simulink model "CH01"  (R2024b)
settings: Solver=FixedStepAuto  StartTime=0.0  StopTime=10  FixedStep=0.001  RelTol=1e-3
settings Model: Creator=headl  LastModifiedBy=headl

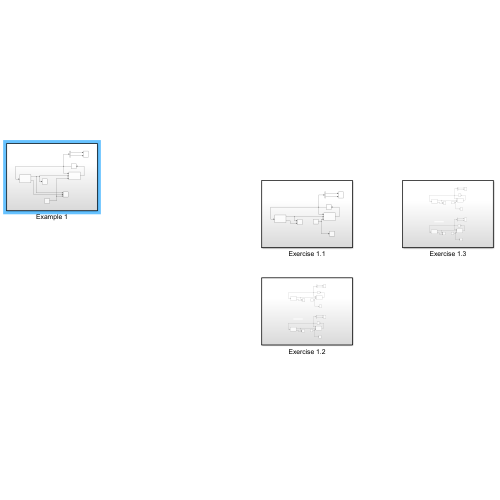
[thumbnail: Simulink's stored preview of the top-level diagram]
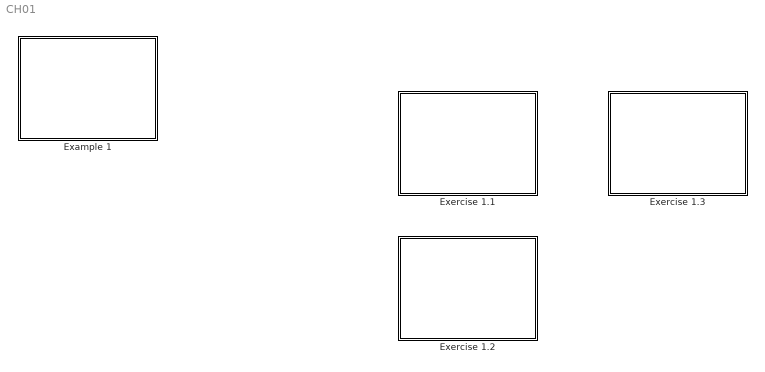
== system CH01 ==
  Example 1 : Subsystem
  Exercise 1.1 : Subsystem
  Exercise 1.2 : Subsystem
  Exercise 1.3 : Subsystem

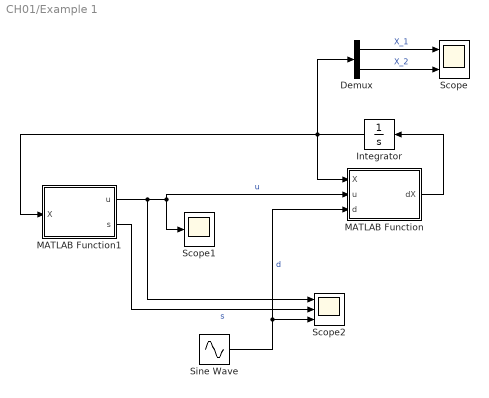
== system CH01/Example 1 ==
  Demux : Demux  Outputs=2
  Integrator : Integrator  InitialCondition=[3;0.4]
  MATLAB Function : MATLAB Function  TreatAsAtomicUnit=on
  MATLAB Function1 : MATLAB Function  TreatAsAtomicUnit=on
  Scope : Scope  NumInputPorts=2
  Scope1 : Scope
  Scope2 : Scope  NumInputPorts=3
  Sine Wave : Sin  Amplitude=0.8  Frequency=4  SampleTime=0
  wires:
  MATLAB Function/1(dX) -> Integrator/1
  Integrator/1 -> Demux/1, MATLAB Function/1(X), MATLAB Function1/1(X)
  Demux/2 -> Scope/2  "X_2"
  MATLAB Function1/1(u) -> Scope2/1, Scope1/1, MATLAB Function/2(u)  "u"
  Demux/1 -> Scope/1  "X_1"
  MATLAB Function1/2(s) -> Scope2/2  "s"
  Sine Wave/1 -> MATLAB Function/3(d), Scope2/3  "d"

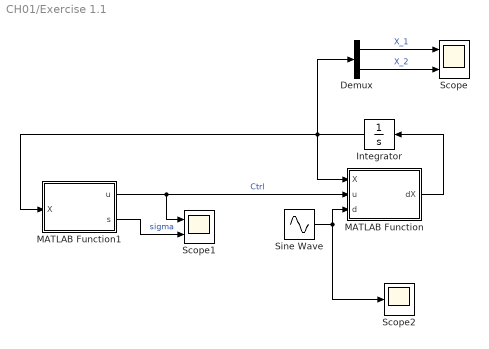
== system CH01/Exercise 1.1 ==
  Demux : Demux  Outputs=2
  Integrator : Integrator  InitialCondition=[2;0.5]
  MATLAB Function : MATLAB Function  TreatAsAtomicUnit=on
  MATLAB Function1 : MATLAB Function  TreatAsAtomicUnit=on
  Scope : Scope  NumInputPorts=2
  Scope1 : Scope  NumInputPorts=2
  Scope2 : Scope
  Sine Wave : Sin  Amplitude=0.4  Frequency=2  SampleTime=0
  wires:
  MATLAB Function/1(dX) -> Integrator/1
  Integrator/1 -> Demux/1, MATLAB Function/1(X), MATLAB Function1/1(X)
  Demux/2 -> Scope/2  "X_2"
  MATLAB Function1/1(u) -> Scope1/1, MATLAB Function/2(u)  "Ctrl"
  Sine Wave/1 -> Scope2/1, MATLAB Function/3(d)
  Demux/1 -> Scope/1  "X_1"
  MATLAB Function1/2(s) -> Scope1/2  "sigma"

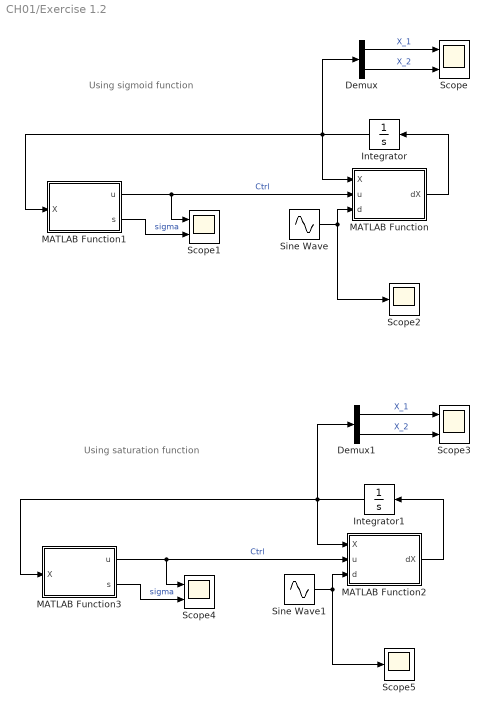
== system CH01/Exercise 1.2 ==
  note: Using sigmoid function
  note: Using saturation function
  Demux : Demux  Outputs=2
  Demux1 : Demux  Outputs=2
  Integrator : Integrator  InitialCondition=[2;0.5]
  Integrator1 : Integrator  InitialCondition=[2;0.5]
  MATLAB Function : MATLAB Function  TreatAsAtomicUnit=on
  MATLAB Function1 : MATLAB Function  TreatAsAtomicUnit=on
  MATLAB Function2 : MATLAB Function  TreatAsAtomicUnit=on
  MATLAB Function3 : MATLAB Function  TreatAsAtomicUnit=on
  Scope{,1,3..4} (4 alike) : Scope  NumInputPorts=2
  Scope2 : Scope
  Scope5 : Scope
  Sine Wave : Sin  Amplitude=0.4  Frequency=2  SampleTime=0
  Sine Wave1 : Sin  Amplitude=0.4  Frequency=2  SampleTime=0
  wires:
  MATLAB Function/1(dX) -> Integrator/1
  Integrator/1 -> Demux/1, MATLAB Function/1(X), MATLAB Function1/1(X)
  Demux/2 -> Scope/2  "X_2"
  MATLAB Function1/1(u) -> Scope1/1, MATLAB Function/2(u)  "Ctrl"
  Sine Wave/1 -> Scope2/1, MATLAB Function/3(d)
  Demux/1 -> Scope/1  "X_1"
  MATLAB Function1/2(s) -> Scope1/2  "sigma"
  Integrator1/1 -> Demux1/1, MATLAB Function2/1(X), MATLAB Function3/1(X)
  MATLAB Function2/1(dX) -> Integrator1/1
  MATLAB Function3/2(s) -> Scope4/2  "sigma"
  Demux1/2 -> Scope3/2  "X_2"
  MATLAB Function3/1(u) -> Scope4/1, MATLAB Function2/2(u)  "Ctrl"
  Demux1/1 -> Scope3/1  "X_1"
  Sine Wave1/1 -> Scope5/1, MATLAB Function2/3(d)

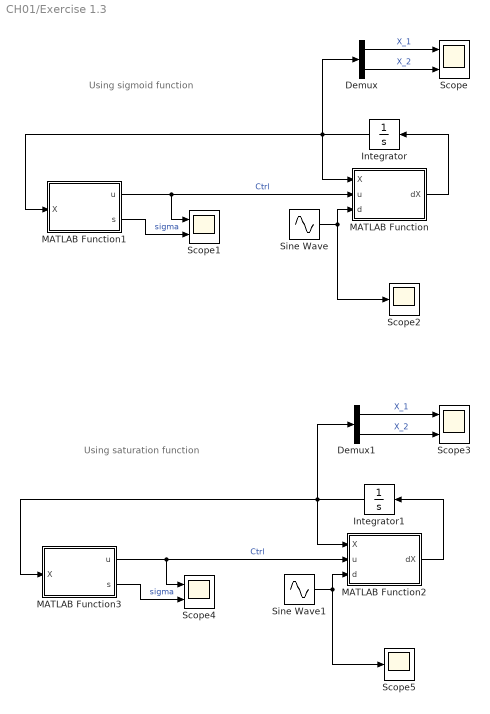
== system CH01/Exercise 1.3 ==
  note: Using sigmoid function
  note: Using saturation function
  Demux : Demux  Outputs=2
  Demux1 : Demux  Outputs=2
  Integrator : Integrator  InitialCondition=[2;0.5]
  Integrator1 : Integrator  InitialCondition=[2;0.5]
  MATLAB Function : MATLAB Function  TreatAsAtomicUnit=on
  MATLAB Function1 : MATLAB Function  TreatAsAtomicUnit=on
  MATLAB Function2 : MATLAB Function  TreatAsAtomicUnit=on
  MATLAB Function3 : MATLAB Function  TreatAsAtomicUnit=on
  Scope{,1,3..4} (4 alike) : Scope  NumInputPorts=2
  Scope2 : Scope
  Scope5 : Scope
  Sine Wave : Sin  Amplitude=0.4  Frequency=2  SampleTime=0
  Sine Wave1 : Sin  Amplitude=0.4  Frequency=2  SampleTime=0
  wires:
  MATLAB Function/1(dX) -> Integrator/1
  Integrator/1 -> Demux/1, MATLAB Function/1(X), MATLAB Function1/1(X)
  Demux/2 -> Scope/2  "X_2"
  MATLAB Function1/1(u) -> Scope1/1, MATLAB Function/2(u)  "Ctrl"
  Sine Wave/1 -> Scope2/1, MATLAB Function/3(d)
  Demux/1 -> Scope/1  "X_1"
  MATLAB Function1/2(s) -> Scope1/2  "sigma"
  Integrator1/1 -> Demux1/1, MATLAB Function2/1(X), MATLAB Function3/1(X)
  MATLAB Function2/1(dX) -> Integrator1/1
  MATLAB Function3/2(s) -> Scope4/2  "sigma"
  Demux1/2 -> Scope3/2  "X_2"
  MATLAB Function3/1(u) -> Scope4/1, MATLAB Function2/2(u)  "Ctrl"
  Demux1/1 -> Scope3/1  "X_1"
  Sine Wave1/1 -> Scope5/1, MATLAB Function2/3(d)

== matlab function CH01/Example 1/MATLAB Function1 ==
  data: X input; u output; s output
function [u, s] = ctrl(X)
k_1 = 2;
k_2 = 3;


c = 3;

rho = 4;
%u = -k_1*X(1) -k_2*X(2);

s = X(2) + c*X(1);
u = -rho*sign(s);

== matlab function CH01/Exercise 1.1/MATLAB Function ==
  data: X input; u input; dX output; d input
function dX = system(X,u,d)
dX = [0;0];
k = 1.5 + d; % d is the disturbance
m = 4;

dX(1) = X(2);

dX(2)= -k*X(2)*abs(X(2)) + u;
dX(2)=dX(2)/m;

== matlab function CH01/Exercise 1.2/MATLAB Function ==
  data: X input; u input; dX output; d input
function dX = system(X,u,d)
dX = [0;0];
k = 1.5 + d; % d is the disturbance
m = 4;

dX(1) = X(2);

dX(2)= -k*X(2)*abs(X(2)) + u;
dX(2)=dX(2)/m;

== matlab function CH01/Exercise 1.2/MATLAB Function1 ==
  data: X input; u output; s output
function [u,s] = ctrl(X)
m = 4;
k_1 = 1.5;
L = 0.8;
c = 3;


k_2 = m/c;
alpha = 3;
s = X(1)+ c*X(2);
rho = L + alpha/sqrt(2);
v = -rho*sigmoid(s,0.01);
u = k_1*X(2)*abs(X(2)) - k_2*X(2)^2 +k_2*v;

end

function z = sigmoid(sigma, epsilon)
    z = sigma / (abs(sigma)+epsilon)
end

== matlab function CH01/Exercise 1.2/MATLAB Function2 ==
  data: X input; u input; dX output; d input
function dX = system(X,u,d)
dX = [0;0];
k = 1.5 + d; % d is the disturbance
m = 4;

dX(1) = X(2);

dX(2)= -k*X(2)*abs(X(2)) + u;
dX(2)=dX(2)/m;

== matlab function CH01/Exercise 1.2/MATLAB Function3 ==
  data: X input; u output; s output
function [u,s] = ctrl(X)
m = 4;
k_1 = 1.5;
L = 0.8;
c = 3;


k_2 = m/c;
alpha = 3;
s = X(1)+ c*X(2);
rho = L + alpha/sqrt(2);
v = -rho*sign2(s,0.01);
u = k_1*X(2)*abs(X(2)) - k_2*X(2)^2 +k_2*v;

end



function z = sign2(sigma, epsilon)
    if sigma > epsilon
        z = 1;
    elseif sigma < -epsilon
        z = -1;
    else
        z = sigma/epsilon;
    end
end

== matlab function CH01/Exercise 1.3/MATLAB Function ==
  data: X input; u input; dX output; d input
function dX = system(X,u,d)
dX = [0;0];
k = 1.5 + d; % d is the disturbance
m = 4;

dX(1) = X(2);

dX(2)= -k*X(2)*abs(X(2)) + u;
dX(2)=dX(2)/m;

== matlab function CH01/Exercise 1.3/MATLAB Function1 ==
  data: X input; u output; s output
function [u,s] = ctrl(X)
m = 4;
k_1 = 1.5;
L = 0.8;
c = 3;


k_2 = m/c;
alpha = 3;
s = X(1)+ c*X(2);
rho = L + alpha/sqrt(2);
v = -rho*sigmoid(s,0.01);
u = k_1*X(2)*abs(X(2)) - k_2*X(2)^2 +k_2*v;

end

function z = sigmoid(sigma, epsilon)
    z = sigma / (abs(sigma)+epsilon)
end

== matlab function CH01/Exercise 1.3/MATLAB Function2 ==
  data: X input; u input; dX output; d input
function dX = system(X,u,d)
dX = [0;0];
k = 1.5 + d; % d is the disturbance
m = 4;

dX(1) = X(2);

dX(2)= -k*X(2)*abs(X(2)) + u;
dX(2)=dX(2)/m;

== matlab function CH01/Exercise 1.3/MATLAB Function3 ==
  data: X input; u output; s output
function [u,s] = ctrl(X)
m = 4;
k_1 = 1.5;
L = 0.8;
c = 3;


k_2 = m/c;
alpha = 3;
s = X(1)+ c*X(2);
rho = L + alpha/sqrt(2);
v = -rho*sign2(s,0.01);
u = k_1*X(2)*abs(X(2)) - k_2*X(2)^2 +k_2*v;

end



function z = sign2(sigma, epsilon)
    if sigma > epsilon
        z = 1;
    elseif sigma < -epsilon
        z = -1;
    else
        z = sigma/epsilon;
    end
end

== matlab function CH01/Exercise 1.1/MATLAB Function1 ==
  data: X input; u output; s output
function [u,s] = ctrl(X)
m = 4;
k_1 = 1.5;
L = 0.8;
c = 3;


k_2 = m/c;
alpha = 3;
s = X(1)+ c*X(2);
rho = L + alpha/sqrt(2);
v = -rho*sign(s);
u = k_1*X(2)*abs(X(2)) - k_2*X(2)^2 +k_2*v;

== matlab function CH01/Example 1/MATLAB Function ==
  data: X input; u input; dX output; d input
function dX = system(X,u,d)
dX = [0;0];
% d is the disturbance

dX(1) = X(2);
dX(2)= u + d;
